simulink model "motor_position_control"  (R2020b)
settings: Solver=VariableStepAuto  StartTime=0.0  StopTime=10.0  RelTol=1e-3
values from neighbouring files (symbols this model uses):
  b = 3.5077e-6    (= 3.5077e-06)    [variable_declaration.m]
  J = 3.2284e-6    (= 3.2284e-06)    [variable_declaration.m]
  kd = 1    [variable_declaration.m]
  Ke = 0.0274    [variable_declaration.m]
  ki = 1    [variable_declaration.m]
  kp = 1    [variable_declaration.m]
  Kt = 0.0274    [variable_declaration.m]
  L = 2.75e-6    (= 2.75e-06)    [variable_declaration.m]
  R = 4    [variable_declaration.m]
settings Model: Creator=shraddha  LastModifiedBy=shraddha

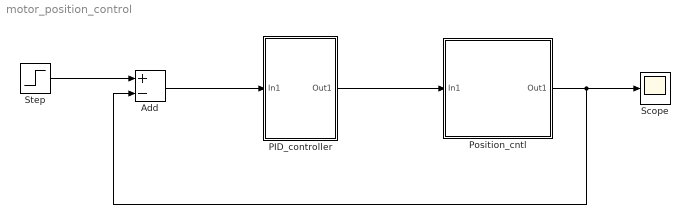
== system motor_position_control ==
  Add : Sum  Inputs=+-
  PID_controller : Subsystem
  Position_cntl : Subsystem
  Scope : Scope
  Step : Step  SampleTime=0
  wires:
  Position_cntl/1(Out1) -> Scope/1, Add/2
  Step/1 -> Add/1
  Add/1 -> PID_controller/1(In1)
  PID_controller/1(Out1) -> Position_cntl/1(In1)

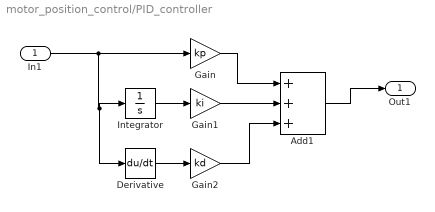
== system motor_position_control/PID_controller ==
  In1 : Inport
  Add1 : Sum  Inputs=+++
  Derivative : Derivative
  Gain : Gain  Gain=kp
  Gain1 : Gain  Gain=ki
  Gain2 : Gain  Gain=kd
  Integrator : Integrator
  Out1 : Outport
  wires:
  Integrator/1 -> Gain1/1
  Gain/1 -> Add1/1
  Gain1/1 -> Add1/2
  In1/1 -> Derivative/1, Integrator/1, Gain/1
  Add1/1 -> Out1/1
  Derivative/1 -> Gain2/1
  Gain2/1 -> Add1/3

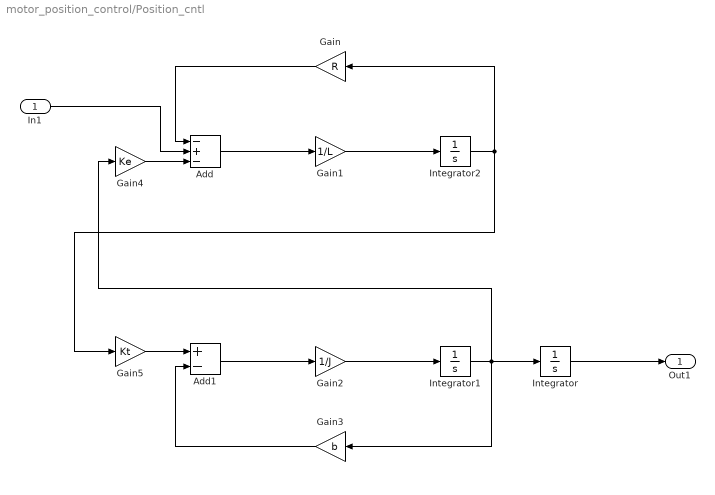
== system motor_position_control/Position_cntl ==
  In1 : Inport
  Add : Sum  Inputs=-+-
  Add1 : Sum  Inputs=+-
  Gain : Gain  Gain=R
  Gain1 : Gain  Gain=1/L
  Gain2 : Gain  Gain=1/J
  Gain3 : Gain  Gain=b
  Gain4 : Gain  Gain=Ke
  Gain5 : Gain  Gain=Kt
  Integrator : Integrator
  Integrator1 : Integrator
  Integrator2 : Integrator
  Out1 : Outport
  wires:
  Integrator1/1 -> Gain4/1, Gain3/1, Integrator/1
  Gain4/1 -> Add/3
  Gain2/1 -> Integrator1/1
  Add1/1 -> Gain2/1
  Gain3/1 -> Add1/2
  Gain1/1 -> Integrator2/1
  Integrator2/1 -> Gain5/1, Gain/1
  Integrator/1 -> Out1/1
  Add/1 -> Gain1/1
  Gain5/1 -> Add1/1
  Gain/1 -> Add/1
  In1/1 -> Add/2
